simulink model "DM"  (R2020a)
settings: Solver=VariableStepAuto  StartTime=0.0  StopTime=10.0  RelTol=1e-3
libraries: dspquant2 x2, dsparch4 x1
settings Model: Creator=koutras  LastModifiedBy=koutras

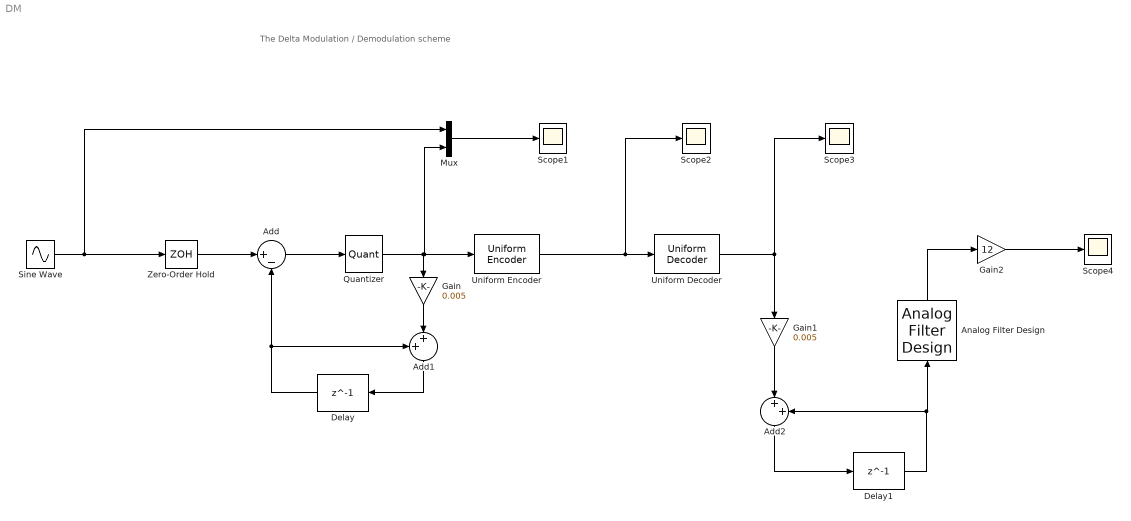
== system DM ==
  note: The Delta Modulation / Demodulation scheme
  Add : Sum  Inputs=|+-
  Add1 : Sum  Inputs=++|
  Add2 : Sum  Inputs=|++
  Analog Filter Design : dsparch4/Analog Filter Design  method=Butterworth  filttype=Lowpass  N=8  Wlo=2*pi*100  Whi=80  Rp=2  Rs=40
  Delay : Delay  DelayLength=1  InitialCondition=0  UseCircularBuffer=on
  Delay1 : Delay  DelayLength=1  InitialCondition=0  UseCircularBuffer=on
  Gain : Gain  Gain=0.005
  Gain1 : Gain  Gain=0.005
  Gain2 : Gain  Gain=12
  Mux : Mux  Inputs=2
  Quantizer : Quantizer  LinearizeAsGain=off
  Scope{1..4} (4 alike) : Scope
  Sine Wave : Sin  Amplitude=1.5  Frequency=2*pi*80  SampleTime=0
  Uniform Decoder : dspquant2/Uniform Decoder  peak=2  bits=8  overflowMode=Saturate  otype=Double
      settings: SourceProductBaseCode=DS
  Uniform Encoder : dspquant2/Uniform Encoder  peak=2  bits=8  otype=Unsigned integer
  Zero-Order Hold : ZeroOrderHold  SampleTime=1/8000
  wires:
  Sine Wave/1 -> Mux/1, Zero-Order Hold/1
  Quantizer/1 -> Uniform Encoder/1, Mux/2, Gain/1
  Zero-Order Hold/1 -> Add/1
  Add/1 -> Quantizer/1
  Delay/1 -> Add/2, Add1/1
  Add1/1 -> Delay/1
  Mux/1 -> Scope1/1
  Uniform Encoder/1 -> Uniform Decoder/1, Scope2/1
  Gain/1 -> Add1/2
  Uniform Decoder/1 -> Gain1/1, Scope3/1
  Gain1/1 -> Add2/1
  Add2/1 -> Delay1/1
  Delay1/1 -> Analog Filter Design/1, Add2/2
  Analog Filter Design/1 -> Gain2/1
  Gain2/1 -> Scope4/1
